simulink model "testBench"  (R2018b)
settings: Solver=VariableStepAuto  StartTime=0.0  StopTime=10.0  RelTol=1e-3
settings Model: Creator=martinandersen  LastModifiedBy=martinandersen

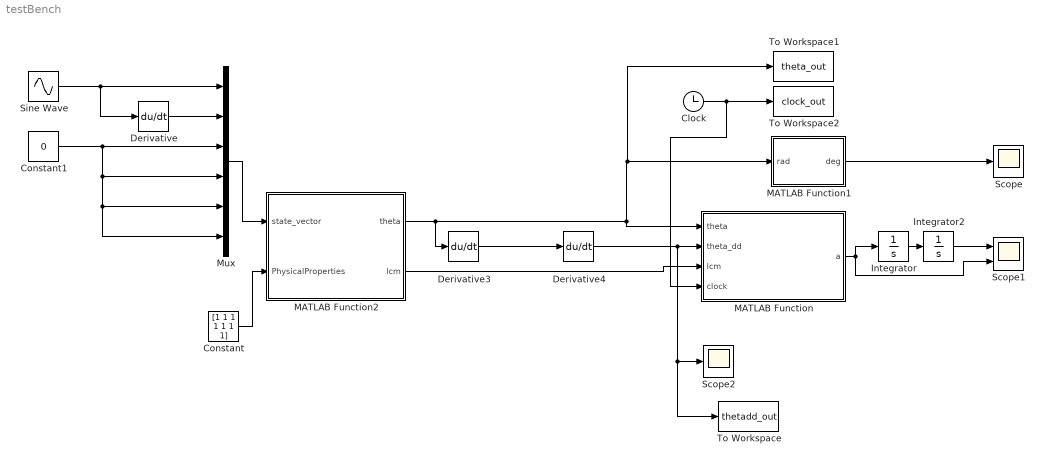
== system testBench ==
  Clock : Clock
  Constant : Constant  Value=[1 1 1 1 1 1 1]
  Constant1 : Constant  Value=0
  Derivative : Derivative
  Derivative3 : Derivative
  Derivative4 : Derivative
  Integrator : Integrator
  Integrator2 : Integrator
  MATLAB Function : MATLAB Function  TreatAsAtomicUnit=on
  MATLAB Function1 : MATLAB Function  TreatAsAtomicUnit=on
  MATLAB Function2 : MATLAB Function  TreatAsAtomicUnit=on
  Mux : Mux  Inputs=6
  Scope : Scope
  Scope1 : Scope  NumInputPorts=2
  Scope2 : Scope
  Sine Wave : Sin  Amplitude=pi/4  SampleTime=0
  To Workspace : ToWorkspace  VariableName=thetadd_out  SaveFormat=Timeseries  SampleTime=-1
  To Workspace1 : ToWorkspace  VariableName=theta_out  SampleTime=-1
  To Workspace2 : ToWorkspace  VariableName=clock_out  SampleTime=-1
  wires:
  MATLAB Function2/2(lcm) -> MATLAB Function/3(lcm)
  MATLAB Function2/1(theta) -> Derivative3/1, To Workspace1/1, MATLAB Function1/1(rad), MATLAB Function/1(theta)
  Integrator/1 -> Integrator2/1
  MATLAB Function/1(a) -> Integrator/1, Scope1/2
  Constant/1 -> MATLAB Function2/2(PhysicalProperties)
  Mux/1 -> MATLAB Function2/1(state_vector)
  Sine Wave/1 -> Derivative/1, Mux/1
  Derivative/1 -> Mux/2
  Constant1/1 -> Mux/6, Mux/5, Mux/4, Mux/3
  Integrator2/1 -> Scope1/1
  MATLAB Function1/1(deg) -> Scope/1
  Derivative4/1 -> Scope2/1, To Workspace/1, MATLAB Function/2(theta_dd)
  Derivative3/1 -> Derivative4/1
  Clock/1 -> MATLAB Function/4(clock), To Workspace2/1

== matlab function testBench/MATLAB Function1 ==
  data: rad input; deg output
function deg = fcn(rad)

deg = rad2deg(rad);

== matlab function testBench/MATLAB Function ==
  data: theta input; a output; theta_dd input; lcm input; clock input
function a = acceleration(theta, theta_dd, lcm, clock)

g = 9.81;

if clock > 0.001
    a = (lcm*theta_dd - g*sin(-theta)) / cos(-theta);
    
else
    a = 0;
end

== matlab function testBench/MATLAB Function2 ==
  data: state_vector input; theta output; PhysicalProperties input; lcm output
function [theta, lcm] = fcn(state_vector, PhysicalProperties)

Theta1 = state_vector(1);
Theta2 = state_vector(3);
Theta3 = state_vector(5);

[cmx, cmz] = CMcalculator(Theta1, Theta2, Theta3, PhysicalProperties);

lcm = sqrt(cmx^2 + cmz^2);


theta = sign(cmx)*acos(cmz/lcm);
